simulink model "Kinematics_Dynamics"  (R2022b)
settings: Solver=VariableStepAuto  StartTime=0.0  StopTime=10.0  RelTol=1e-3
model workspace (MAT data in the model file):
  mass = 1.56
values from neighbouring files (symbols this model uses):
  fx = 10    [Kinematics_Dynamics_Init.m]
  fy = 2    [Kinematics_Dynamics_Init.m]
  fz = 0    [Kinematics_Dynamics_Init.m]
  Jx = 0.1147    [Kinematics_Dynamics_Init.m]
  Jxy = 0    [Kinematics_Dynamics_Init.m]
  Jxz = 0.0015    [Kinematics_Dynamics_Init.m]
  Jy = 0.0576    [Kinematics_Dynamics_Init.m]
  Jyz = 0    [Kinematics_Dynamics_Init.m]
  Jz = 0.1712    [Kinematics_Dynamics_Init.m]
  L = 0.1    [Kinematics_Dynamics_Init.m]
  M = 0    [Kinematics_Dynamics_Init.m]
  N = 0    [Kinematics_Dynamics_Init.m]
  n_e_d_init = [0; 0; 0;]    [Kinematics_Dynamics_Init.m]
  p_q_r_init = [0; 0; 0;]    [Kinematics_Dynamics_Init.m]
  phi_theta_psi_init = [10; 0; 0;]    [Kinematics_Dynamics_Init.m]
  u_v_w_init = [15; 0; 0;]    [Kinematics_Dynamics_Init.m]
  x_y_z_init = [0; 0; 0;]    [Kinematics_Dynamics_Init.m]
libraries: matrix_library x1
settings Model: Creator=Admin  LastModifiedBy=Admin

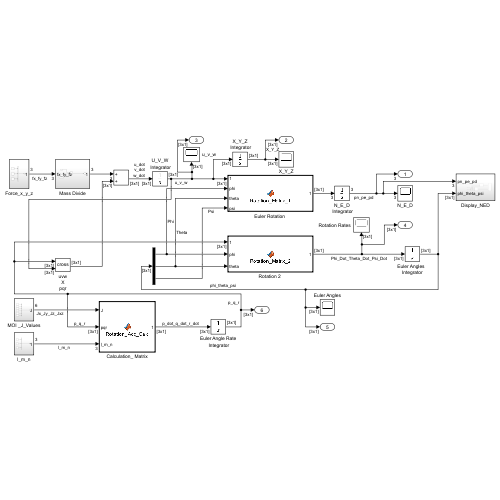
[thumbnail: Simulink's stored preview of the top-level diagram]
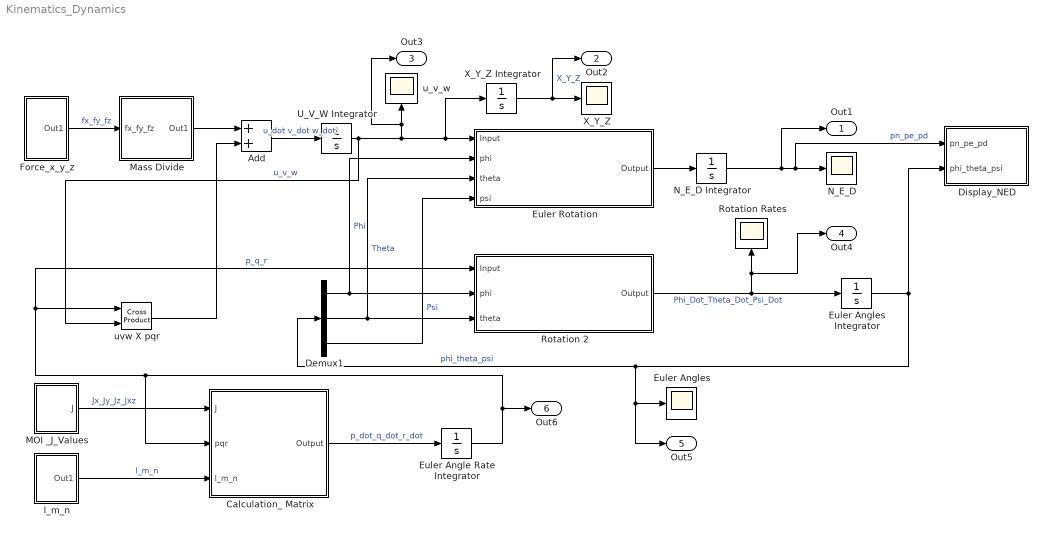
== system Kinematics_Dynamics ==
  Add : Sum
  Calculation_ Matrix : MATLAB Function  TreatAsAtomicUnit=on
  Demux1 : Demux  Outputs=3
  Display_NED : Subsystem
  Euler Angle Rate Integrator : Integrator  InitialCondition=p_q_r_init
  Euler Angles : Scope
  Euler Angles Integrator : Integrator  InitialCondition=phi_theta_psi_init
  "Euler Rotation " : MATLAB Function  TreatAsAtomicUnit=on
  Force_x_y_z : Subsystem
  MOI _J_Values : Subsystem
  Mass Divide : Subsystem
  N_E_D : Scope
  N_E_D Integrator : Integrator  InitialCondition=n_e_d_init
  "Rotation 2 " : MATLAB Function  TreatAsAtomicUnit=on
  Rotation Rates : Scope
  U_V_W Integrator : Integrator  InitialCondition=u_v_w_init
  X_Y_Z : Scope
  X_Y_Z Integrator : Integrator  InitialCondition=x_y_z_init
  l_m_n : Subsystem
  u_v_w : Scope
  uvw X pqr : matrix_library/Cross Product
  Out1 : Outport
  Out2 : Outport  Port=2
  Out3 : Outport  Port=3
  Out4 : Outport  Port=4
  Out5 : Outport  Port=5
  Out6 : Outport  Port=6
  wires:
  U_V_W Integrator/1 -> "Euler Rotation "/1(Input), X_Y_Z Integrator/1, Out3/1, u_v_w/1, uvw X pqr/2  "u_v_w"
  uvw X pqr/1 -> Add/2
  Add/1 -> U_V_W Integrator/1  "u_dot v_dot w_dot"
  "Euler Rotation "/1(Output) -> N_E_D Integrator/1
  N_E_D Integrator/1 -> Out1/1, Display_NED/1(pn_pe_pd), N_E_D/1  "pn_pe_pd"
  "Rotation 2 "/1(Output) -> Rotation Rates/1, Out4/1, Euler Angles Integrator/1  "Phi_Dot_Theta_Dot_Psi_Dot"
  Euler Angles Integrator/1 -> Display_NED/2(phi_theta_psi), Demux1/1, Out5/1, Euler Angles/1  "phi_theta_psi"
  Demux1/2 -> "Euler Rotation "/3(theta), "Rotation 2 "/3(theta)  "Theta"
  Demux1/1 -> "Euler Rotation "/2(phi), "Rotation 2 "/2(phi)  "Phi"
  Demux1/3 -> "Euler Rotation "/4(psi)  "Psi"
  Calculation_ Matrix/1(Output) -> Euler Angle Rate Integrator/1  "p_dot_q_dot_r_dot"
  Euler Angle Rate Integrator/1 -> uvw X pqr/1, "Rotation 2 "/1(Input), Calculation_ Matrix/2(pqr), Out6/1  "p_q_r"
  l_m_n/1(Out1) -> Calculation_ Matrix/3(l_m_n)  "l_m_n"
  MOI _J_Values/1(J) -> Calculation_ Matrix/1(J)  "Jx_Jy_Jz_Jxz"
  X_Y_Z Integrator/1 -> Out2/1, X_Y_Z/1  "X_Y_Z"
  Force_x_y_z/1(Out1) -> Mass Divide/1(fx_fy_fz)  "fx_fy_fz"
  Mass Divide/1(Out1) -> Add/1

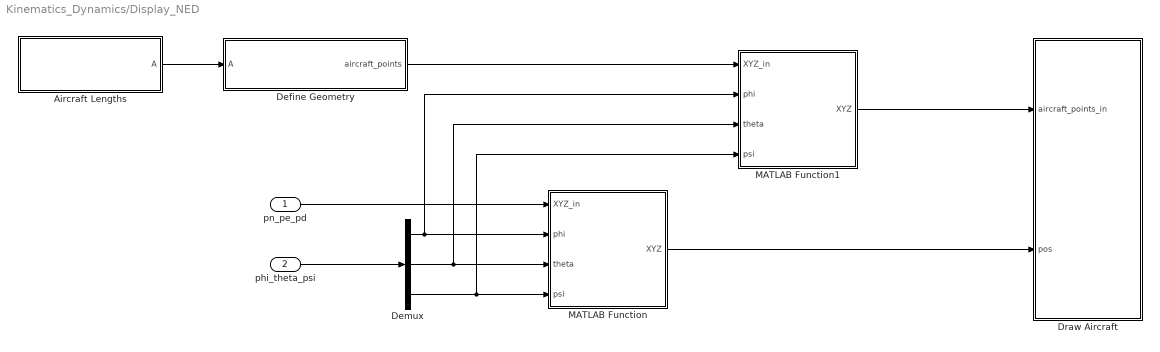
== system Kinematics_Dynamics/Display_NED ==
  pn_pe_pd : Inport
  phi_theta_psi : Inport  Port=2
  Aircraft Lengths : MATLAB Function  TreatAsAtomicUnit=on
  Define Geometry : MATLAB Function  TreatAsAtomicUnit=on
  Demux : Demux  Outputs=3
  Draw Aircraft : MATLAB Function  TreatAsAtomicUnit=on
  MATLAB Function : MATLAB Function  TreatAsAtomicUnit=on
  MATLAB Function1 : MATLAB Function  TreatAsAtomicUnit=on
  wires:
  Aircraft Lengths/1(A) -> Define Geometry/1(A)
  phi_theta_psi/1 -> Demux/1
  Demux/1 -> MATLAB Function1/2(phi), MATLAB Function/2(phi)
  Demux/2 -> MATLAB Function1/3(theta), MATLAB Function/3(theta)
  Demux/3 -> MATLAB Function1/4(psi), MATLAB Function/4(psi)
  pn_pe_pd/1 -> MATLAB Function/1(XYZ_in)
  MATLAB Function/1(XYZ) -> Draw Aircraft/2(pos)
  MATLAB Function1/1(XYZ) -> Draw Aircraft/1(aircraft_points_in)
  Define Geometry/1(aircraft_points) -> MATLAB Function1/1(XYZ_in)

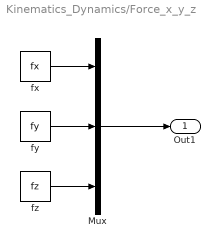
== system Kinematics_Dynamics/Force_x_y_z ==
  Mux : Mux  Inputs=3
  fx : Constant  Value=fx
  fy : Constant  Value=fy
  fz : Constant  Value=fz
  Out1 : Outport
  wires:
  fx/1 -> Mux/1
  fy/1 -> Mux/2
  fz/1 -> Mux/3
  Mux/1 -> Out1/1

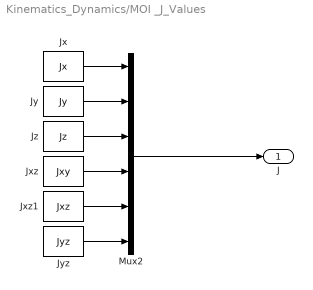
== system Kinematics_Dynamics/MOI _J_Values ==
  Jx : Constant  Value=Jx
  Jxz : Constant  Value=Jxy
  Jxz1 : Constant  Value=Jxz
  Jy : Constant  Value=Jy
  Jyz : Constant  Value=Jyz
  Jz : Constant  Value=Jz
  Mux2 : Mux  Inputs=6
  J : Outport
  wires:
  Jz/1 -> Mux2/3
  Mux2/1 -> J/1
  Jx/1 -> Mux2/1
  Jy/1 -> Mux2/2
  Jxz/1 -> Mux2/4
  Jxz1/1 -> Mux2/5
  Jyz/1 -> Mux2/6

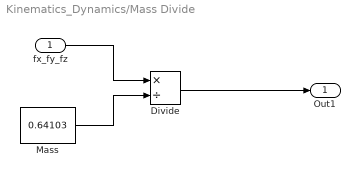
== system Kinematics_Dynamics/Mass Divide ==
  fx_fy_fz : Inport
  Divide : Product  Inputs=*/  RndMeth=Zero  SaturateOnIntegerOverflow=on
  Mass : Constant  Value=0.64103
  Out1 : Outport
  wires:
  fx_fy_fz/1 -> Divide/1
  Mass/1 -> Divide/2
  Divide/1 -> Out1/1

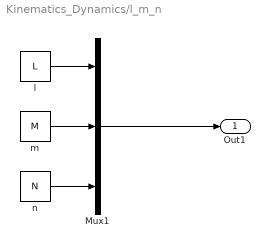
== system Kinematics_Dynamics/l_m_n ==
  Mux1 : Mux  Inputs=3
  l : Constant  Value=L
  m : Constant  Value=M
  n : Constant  Value=N
  Out1 : Outport
  wires:
  n/1 -> Mux1/3
  m/1 -> Mux1/2
  Mux1/1 -> Out1/1
  l/1 -> Mux1/1

== matlab function Kinematics_Dynamics/Rotation 2  ==
  data: Input input; Output output; phi input; theta input
function Output = Rotation_Matrix_2(Input, phi, theta)

R = [1 sind(phi)*tand(theta) cos(phi)*tand(theta);
     0 cosd(phi) -sind(phi);
     0 -sind(phi)*secd(theta) cosd(phi)*secd(theta);];
Output = R*Input;
% set_angles(phi,theta,psi);
end

== matlab function Kinematics_Dynamics/Euler Rotation  ==
  data: Input input; Output output; phi input; theta input; psi input
function Output = Rotation_Matrix_1(Input, phi, theta, psi)
R_roll = [1 0 0;
          0 cosd(phi) sind(phi);
          0 -sind(phi) cosd(phi);];

R_pitch = [cosd(theta) 0 -sind(theta);
           0 1 0;
           sind(theta) 0 cosd(theta);];

R_yaw = [cosd(psi) sind(psi) 0;
         -sind(psi) cosd(psi) 0;
         0 0 1;];

R = R_roll*R_pitch*R_yaw;
Output = (R*Input);
% set_angles(phi,theta,psi);
end

== matlab function Kinematics_Dynamics/Calculation_ Matrix ==
  data: J input; pqr input; Output output; l_m_n input
function Output =  Rotation_Acc_Calc(J, pqr, l_m_n)

R1 = [0 pqr(3) -pqr(2);
      -pqr(3) 0 pqr(1);
      pqr(2) -pqr(1) 0;];
J1 = [J(1) -J(4) -J(5);
      -J(4) J(2) -J(6);
      -J(5) -J(6) J(3);];
pqr1 = [pqr(1);
        pqr(2);
        pqr(3);];
lmn1 = [l_m_n(1);
        l_m_n(2);
        l_m_n(3);];

% if cond(J1) ~= inf
%     J_inv = inv(J1);
% elseif cond(J1) == inf
%     error("MOI Matrix is singular")
% end
J_inv = inv(J1);

% J2 = [J(3)/D 0 J(4)/D;
%       0 1/J(2) 0;
%       J(4)/D 0 J(1)/D];
% 
% temp = R1*J1*pqr1 + lmn1;
Output = J_inv*(R1*J1*pqr1 + lmn1);
end

== matlab function Kinematics_Dynamics/Display_NED/Define Geometry ==
  data: A input; aircraft_points output
function aircraft_points= Def_Geom(A)
%%
% A(1), A(2), A(3), A(4), A(5), A(6), A(7), A(8), A(9), A(10), A(11)
% Matrix A is defined as the order of Aircraft part lengths as given above
% in order of appearnace. A is 11 X 1 Matrix
%%
% Geometry Variables
aircraft_points = [
            A(9), 0, 0; % Point 1
            A(10), A(7)/2, -A(8)/2; % Point 2
            A(10), -A(7)/2, -A(8)/2; % Point 3
            A(10), -A(7)/2, A(8)/2; % Point 4
            A(10), A(7)/2, A(8)/2; % Point 5
            -A(11), 0, 0; % Point 6
            0, A(2)/2, 0; % Point 7
            -A(1), A(2)/2, 0; % Point 8
            -A(1), -A(2)/2, 0; % Point 9
            0, -A(2)/2, 0; % Point 10
            -A(11)+A(3), A(4)/2,0; % Point 11
            -A(11), A(4)/2,0; % Point 12
            -A(11), -A(4)/2,0; % Point 13
            -A(11)+A(3), -A(4)/2,0; % Point 14
            -A(11)+A(6), 0, 0; % Point 15
            -A(11), 0, -A(5); % Point 16
            ];
end

== matlab function Kinematics_Dynamics/Display_NED/Draw Aircraft ==
  data: aircraft_points_in input; pos input
function Draw_Aircraft(aircraft_points_in, pos)
aircraft_faces3 = [
            1 2 3; % Nose
            1 2 5; % Nose
            1 4 5; % Nose
            1 3 4; % Nose
            2 3 6; % Fuselage
            3 4 6; % Fuselage
            4 5 6; % Fuselage
            2 5 6; % Fuselage
            15 16 6; % Vertical Tail
            ];
aircraft_faces4 = [
            7 8 9 10; % Wing
            11 12 13 14; % Horizontal Tail
            2 3 4 5; % Nose-Fuselage
            ];


hold on
figure(1)
cla
rows = size(aircraft_points_in',1);
move = [repelem(pos(1),rows);repelem(pos(2),rows);repelem(pos(3),rows);]';
aircraft_points = aircraft_points_in' + move;
patch('Faces', aircraft_faces3,'Vertices', aircraft_points,'FaceColor', 'red')
patch('Faces', aircraft_faces4,'Vertices', aircraft_points,'FaceColor', 'blue')
xlabel("X-Label")
ylabel("Y-Label")
zlabel("Z-Label")
set(gca,"ZDir",'reverse')
axis equal
grid on
end

== matlab function Kinematics_Dynamics/Display_NED/Aircraft Lengths ==
  data: A output
function A = Aircraft_lengths()
aircraft_lengths = [2 20 1 6 1.5 1.5 1.5 1.5 4 2 15];
A = aircraft_lengths;
end

== matlab function Kinematics_Dynamics/Display_NED/MATLAB Function ==
  data: XYZ_in input; XYZ output; phi input; theta input; psi input
function XYZ = rotate(XYZ_in, phi, theta, psi)
R_roll = [1 0 0;
          0 cosd(phi) sind(phi);
          0 -sind(phi) cosd(phi);];

R_pitch = [cosd(theta) 0 -sind(theta);
           0 1 0;
           sind(theta) 0 cosd(theta);];

R_yaw = [cosd(psi) sind(psi) 0;
         -sind(psi) cosd(psi) 0;
         0 0 1;];

R = R_roll*R_pitch*R_yaw;
XYZ = (R*XYZ_in);

== matlab function Kinematics_Dynamics/Display_NED/MATLAB Function1 ==
  data: XYZ_in input; XYZ output; phi input; theta input; psi input
function XYZ = rotate(XYZ_in , phi, theta, psi)
R_roll = [1 0 0;
          0 cosd(phi) sind(phi);
          0 -sind(phi) cosd(phi);];

R_pitch = [cosd(theta) 0 -sind(theta);
           0 1 0;
           sind(theta) 0 cosd(theta);];

R_yaw = [cosd(psi) sind(psi) 0;
         -sind(psi) cosd(psi) 0;
         0 0 1;];

R = R_roll*R_pitch*R_yaw;
XYZ = (R*XYZ_in');
